simulink model "capstone_sim"  (R2021a)
settings: Solver=VariableStepAuto  StartTime=0.0  StopTime=1.5  RelTol=1e-3
values from neighbouring files (symbols this model uses):
  Jm = 500*(10^-3)*(10^-2)^2    (= 5e-05)    [capstone.m]
  Ka_cur = 1/Kp_cur    (= 521477.533066)    [capstone.m]
  Ka_spd = 1/Kp_spd    (= 8.45112747818)    [capstone.m]
  Kd_pos = Wcp/Wcs    (= 0.1)    [capstone.m]
  Ke = 0.0531    [capstone.m]
  Ki_cur = Ra * Wcc    (= 273.946879393)    [capstone.m]
  Ki_spd = Kp_spd*Wcs/5    (= 2.97389209826)    [capstone.m]
  Kp_cur = La * Wcc    (= 1.91762815575e-06)    [capstone.m]
  Kp_pos = Wcp    (= 12.5663706144)    [capstone.m]
  Kp_spd = Jm*Wcs/Ke    (= 0.118327406915)    [capstone.m]
  Kt = 0.0531    [capstone.m]
  La = 1.526*10^-9    (= 1.526e-09)    [capstone.m]
  Loadtorq = m*9.81*0.01/20    (= 0)    [capstone.m]
  max_cur = 12    [capstone.m]
  max_spd = 3000*(30/pi)    (= 28647.8897565)    [capstone.m]
  n = 20    [capstone.m]
  Ra = 0.218    [capstone.m]
  tau = 1    [capstone.m]
  wa = 10    [capstone.m]
settings Model: PacingRate=1000  Creator=syl12  LastModifiedBy=syl12

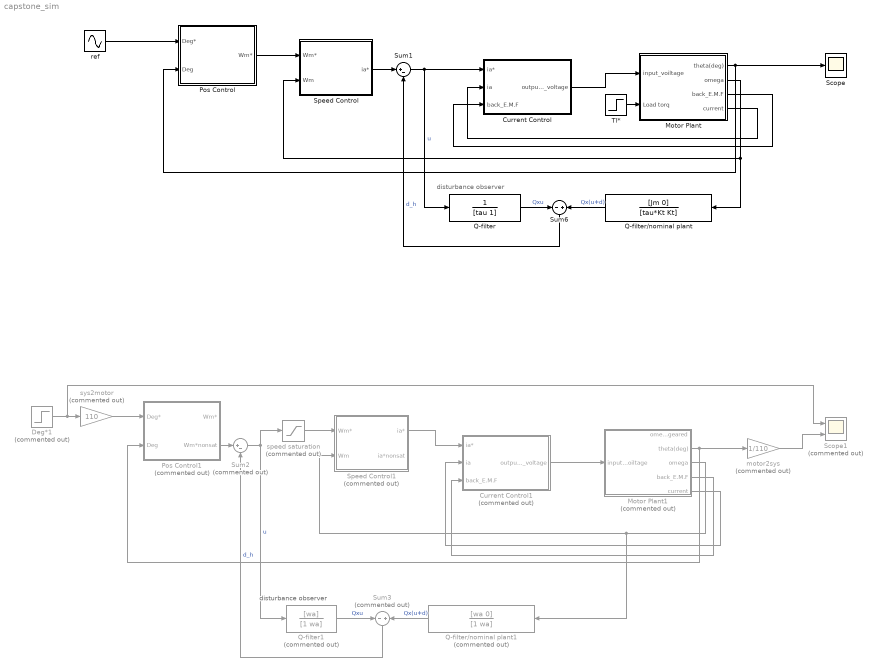
== system capstone_sim ==
  note: disturbance observer
  note: disturbance observer
  Current Control : Subsystem
  Current Control1 : Subsystem  Commented=on
  Deg*1 : Step  Commented=on  Time=0  After=5  SampleTime=0
  Motor Plant : Subsystem
  Motor Plant1 : Subsystem  Commented=on
  Pos Control : Subsystem
  Pos Control1 : Subsystem  Commented=on
  Q-filter : TransferFcn  Denominator=[tau 1]
  Q-filter/nominal plant : TransferFcn  Numerator=[Jm 0]  Denominator=[tau*Kt Kt]
  Q-filter/nominal plant1 : TransferFcn  Commented=on  Numerator=[wa 0]  Denominator=[1 wa]
  Q-filter1 : TransferFcn  Commented=on  Numerator=[wa]  Denominator=[1 wa]
  Scope : Scope
  Scope1 : Scope  Commented=on  NumInputPorts=2
  Speed Control : Subsystem
  Speed Control1 : Subsystem  Commented=on
  Sum1 : Sum  Inputs=|+-
  Sum2 : Sum  Commented=on  Inputs=|+-
  Sum3 : Sum  Commented=on  Inputs=-|+
  Sum6 : Sum  Inputs=-|+
  Tl* : Step  Time=0  After=5  SampleTime=0
  motor2sys : Gain  Commented=on  Gain=1/110
  ref : Sin  Amplitude=5  Frequency=0.15915  SampleTime=0
  speed saturation : Saturate  Commented=on  UpperLimit=max_spd*60/(2*pi*20)  LowerLimit=-max_spd*60/(2*pi*20)
  sys2motor : Gain  Commented=on  Gain=110
  wires:
  Pos Control/1(Wm*) -> Speed Control/1(Wm*)
  Speed Control/1(ia*) -> Sum1/1
  Motor Plant/4(current) -> Current Control/2(ia)
  Motor Plant/2(omega) -> Speed Control/2(Wm), Q-filter/nominal plant/1
  Motor Plant/3(back_E.M.F) -> Current Control/3(back_E.M.F)
  Q-filter/nominal plant/1 -> Sum6/2  "Qx(u+d)"
  Sum1/1 -> Current Control/1(ia*), Q-filter/1  "u"
  Current Control/1(output_voltage) -> Motor Plant/1(input_voiltage)
  Q-filter/1 -> Sum6/1  "Qxu"
  ref/1 -> Pos Control/1(Deg*)
  Motor Plant/1(theta(deg)) -> Scope/1, Pos Control/2(Deg)
  motor2sys/1 -> Scope1/2
  sys2motor/1 -> Pos Control1/1(Deg*)
  Motor Plant1/4(back_E.M.F) -> Current Control1/3(back_E.M.F)
  Motor Plant1/2(theta(deg)) -> motor2sys/1, Pos Control1/2(Deg)
  Motor Plant1/3(omega) -> Q-filter/nominal plant1/1, Speed Control1/2(Wm)
  Deg*1/1 -> Scope1/1, sys2motor/1
  Speed Control1/1(ia*) -> Current Control1/1(ia*)
  Motor Plant1/5(current) -> Current Control1/2(ia)
  Current Control1/1(output_voltage) -> Motor Plant1/1(input_voiltage)
  Q-filter/nominal plant1/1 -> Sum3/2  "Qx(u+d)"
  Q-filter1/1 -> Sum3/1  "Qxu"
  Pos Control1/2(Wm*nonsat) -> Sum2/1
  speed saturation/1 -> Speed Control1/1(Wm*)
  Sum2/1 -> speed saturation/1, Q-filter1/1  "u"
  Sum3/1 -> Sum2/2  "d_h"
  Sum6/1 -> Sum1/2  "d_h"
  Tl*/1 -> Motor Plant/2(Load torq)

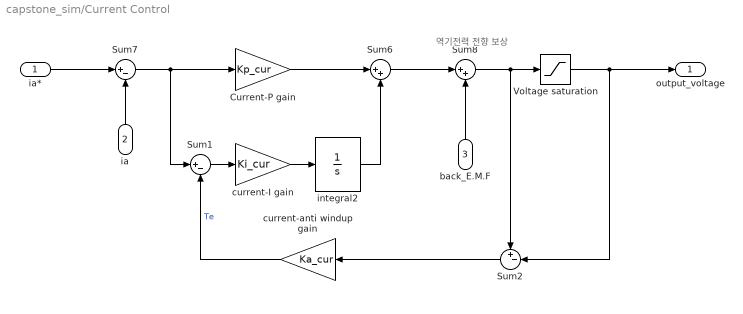
== system capstone_sim/Current Control ==
  note: 역기전력 전향 보상
  ia* : Inport
  ia : Inport  Port=2
  back_E.M.F : Inport  Port=3
  Current-P gain : Gain  Gain=Kp_cur
  Sum1 : Sum  Inputs=|+-
  Sum2 : Sum  Inputs=+-|
  Sum6 : Sum  Inputs=|++
  Sum7 : Sum  Inputs=|+-
  Sum8 : Sum  Inputs=|++
  Voltage saturation : Saturate  UpperLimit=24  LowerLimit=-24  ZeroCross=off
  current-I gain : Gain  Gain=Ki_cur
  current-anti windup gain : Gain  Gain=Ka_cur
  integral2 : TransferFcn  Denominator=[1 0]
  output_voltage : Outport
  wires:
  Sum6/1 -> Sum8/1
  ia*/1 -> Sum7/1
  integral2/1 -> Sum6/2
  Sum7/1 -> Current-P gain/1, Sum1/1
  Current-P gain/1 -> Sum6/1
  current-I gain/1 -> integral2/1
  back_E.M.F/1 -> Sum8/2
  Voltage saturation/1 -> Sum2/2, output_voltage/1
  Sum8/1 -> Sum2/1, Voltage saturation/1
  ia/1 -> Sum7/2
  Sum1/1 -> current-I gain/1
  current-anti windup gain/1 -> Sum1/2  "Te"
  Sum2/1 -> current-anti windup gain/1

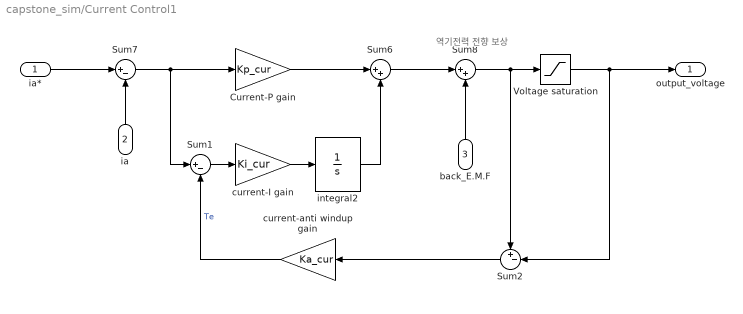
== system capstone_sim/Current Control1 ==
  note: 역기전력 전향 보상
  ia* : Inport
  ia : Inport  Port=2
  back_E.M.F : Inport  Port=3
  Current-P gain : Gain  Gain=Kp_cur
  Sum1 : Sum  Inputs=|+-
  Sum2 : Sum  Inputs=+-|
  Sum6 : Sum  Inputs=|++
  Sum7 : Sum  Inputs=|+-
  Sum8 : Sum  Inputs=|++
  Voltage saturation : Saturate  UpperLimit=24  LowerLimit=-24  ZeroCross=off
  current-I gain : Gain  Gain=Ki_cur
  current-anti windup gain : Gain  Gain=Ka_cur
  integral2 : TransferFcn  Denominator=[1 0]
  output_voltage : Outport
  wires:
  Sum6/1 -> Sum8/1
  ia*/1 -> Sum7/1
  integral2/1 -> Sum6/2
  Sum7/1 -> Current-P gain/1, Sum1/1
  Current-P gain/1 -> Sum6/1
  current-I gain/1 -> integral2/1
  back_E.M.F/1 -> Sum8/2
  Voltage saturation/1 -> Sum2/2, output_voltage/1
  Sum8/1 -> Sum2/1, Voltage saturation/1
  ia/1 -> Sum7/2
  Sum1/1 -> current-I gain/1
  current-anti windup gain/1 -> Sum1/2  "Te"
  Sum2/1 -> current-anti windup gain/1

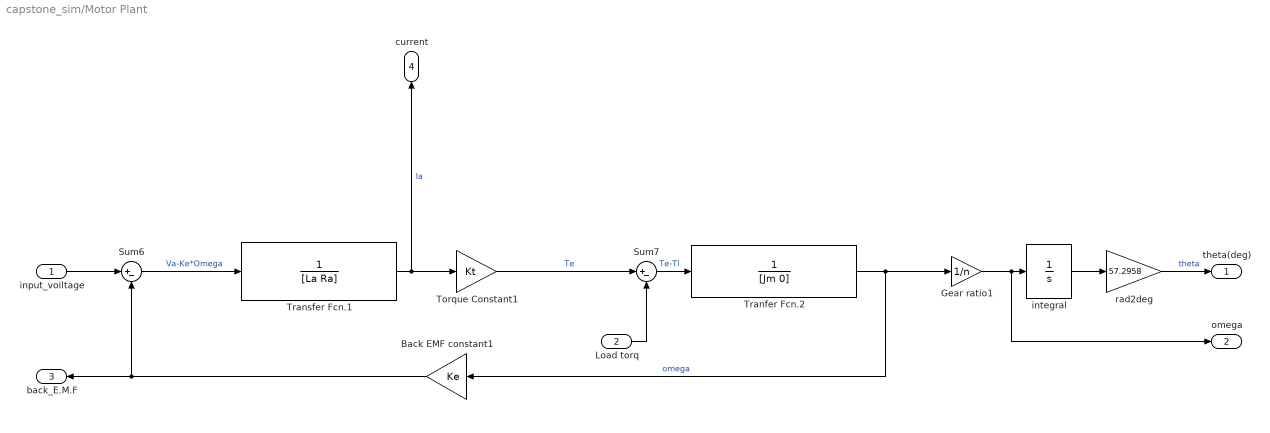
== system capstone_sim/Motor Plant ==
  input_voiltage : Inport
  Load torq : Inport  Port=2
  Back EMF constant1 : Gain  Gain=Ke
  Gear ratio1 : Gain  Gain=1/n
  Sum6 : Sum  Inputs=|+-
  Sum7 : Sum  Inputs=|+-
  Torque Constant1 : Gain  Gain=Kt
  Tranfer Fcn.2 : TransferFcn  Denominator=[Jm 0]
  Transfer Fcn.1 : TransferFcn  Denominator=[La Ra]
  integral : TransferFcn  Denominator=[1 0]
  rad2deg : Gain  Gain=57.2958
  theta(deg) : Outport
  omega : Outport  Port=2
  back_E.M.F : Outport  Port=3
  current : Outport  Port=4
  wires:
  Sum6/1 -> Transfer Fcn.1/1  "Va-Ke*Omega"
  Tranfer Fcn.2/1 -> Gear ratio1/1, Back EMF constant1/1  "omega"
  Sum7/1 -> Tranfer Fcn.2/1  "Te-Tl"
  Back EMF constant1/1 -> back_E.M.F/1, Sum6/2
  input_voiltage/1 -> Sum6/1
  Transfer Fcn.1/1 -> Torque Constant1/1, current/1  "Ia"
  integral/1 -> rad2deg/1
  rad2deg/1 -> theta(deg)/1  "theta"
  Gear ratio1/1 -> omega/1, integral/1
  Torque Constant1/1 -> Sum7/1  "Te"
  Load torq/1 -> Sum7/2

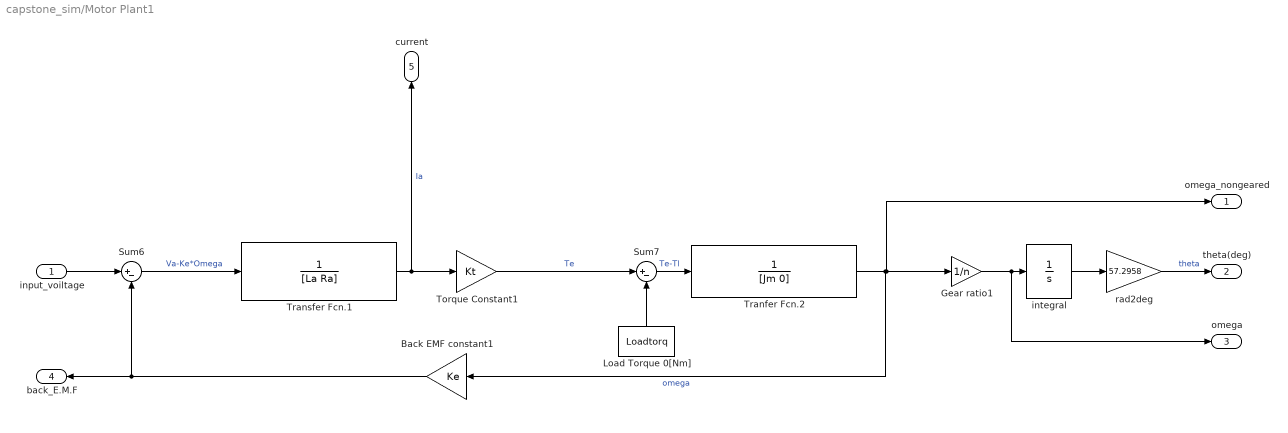
== system capstone_sim/Motor Plant1 ==
  input_voiltage : Inport
  Back EMF constant1 : Gain  Gain=Ke
  Gear ratio1 : Gain  Gain=1/n
  Load Torque 0[Nm] : Constant  Value=Loadtorq
  Sum6 : Sum  Inputs=|+-
  Sum7 : Sum  Inputs=|+-
  Torque Constant1 : Gain  Gain=Kt
  Tranfer Fcn.2 : TransferFcn  Denominator=[Jm 0]
  Transfer Fcn.1 : TransferFcn  Denominator=[La Ra]
  integral : TransferFcn  Denominator=[1 0]
  rad2deg : Gain  Gain=57.2958
  omega_nongeared : Outport
  theta(deg) : Outport  Port=2
  omega : Outport  Port=3
  back_E.M.F : Outport  Port=4
  current : Outport  Port=5
  wires:
  Sum6/1 -> Transfer Fcn.1/1  "Va-Ke*Omega"
  Tranfer Fcn.2/1 -> omega_nongeared/1, Gear ratio1/1, Back EMF constant1/1  "omega"
  Sum7/1 -> Tranfer Fcn.2/1  "Te-Tl"
  Back EMF constant1/1 -> back_E.M.F/1, Sum6/2
  input_voiltage/1 -> Sum6/1
  Transfer Fcn.1/1 -> Torque Constant1/1, current/1  "Ia"
  integral/1 -> rad2deg/1
  rad2deg/1 -> theta(deg)/1  "theta"
  Gear ratio1/1 -> omega/1, integral/1
  Torque Constant1/1 -> Sum7/1  "Te"
  Load Torque 0[Nm]/1 -> Sum7/2

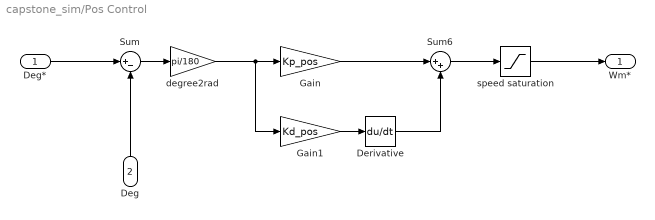
== system capstone_sim/Pos Control ==
  Deg* : Inport
  Deg : Inport  Port=2
  Derivative : Derivative
  Gain : Gain  Gain=Kp_pos
  Gain1 : Gain  Gain=Kd_pos
  Sum : Sum  Inputs=|+-
  Sum6 : Sum  Inputs=|++
  degree2rad : Gain  Gain=pi/180
  speed saturation : Saturate  UpperLimit=max_spd*60/(2*pi*20)  LowerLimit=-max_spd*60/(2*pi*20)
  Wm* : Outport
  wires:
  Derivative/1 -> Sum6/2
  Deg*/1 -> Sum/1
  speed saturation/1 -> Wm*/1
  Gain/1 -> Sum6/1
  Sum6/1 -> speed saturation/1
  Deg/1 -> Sum/2
  Gain1/1 -> Derivative/1
  Sum/1 -> degree2rad/1
  degree2rad/1 -> Gain1/1, Gain/1

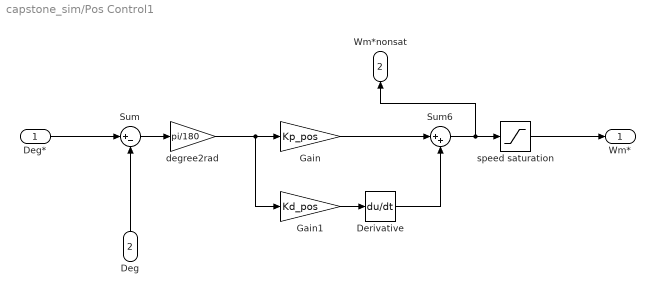
== system capstone_sim/Pos Control1 ==
  Deg* : Inport
  Deg : Inport  Port=2
  Derivative : Derivative
  Gain : Gain  Gain=Kp_pos
  Gain1 : Gain  Gain=Kd_pos
  Sum : Sum  Inputs=|+-
  Sum6 : Sum  Inputs=|++
  degree2rad : Gain  Gain=pi/180
  speed saturation : Saturate  UpperLimit=max_spd*60/(2*pi*20)  LowerLimit=-max_spd*60/(2*pi*20)
  Wm* : Outport
  Wm*nonsat : Outport  Port=2
  wires:
  Derivative/1 -> Sum6/2
  Deg*/1 -> Sum/1
  speed saturation/1 -> Wm*/1
  Gain/1 -> Sum6/1
  Sum6/1 -> speed saturation/1, Wm*nonsat/1
  Deg/1 -> Sum/2
  Gain1/1 -> Derivative/1
  Sum/1 -> degree2rad/1
  degree2rad/1 -> Gain1/1, Gain/1

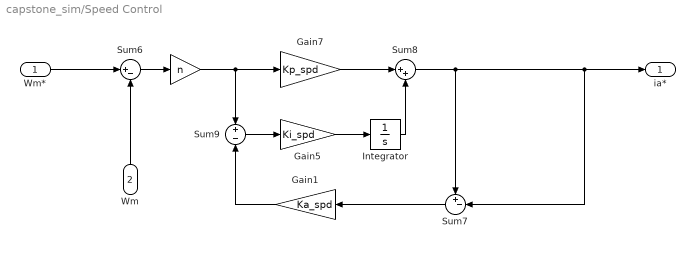
== system capstone_sim/Speed Control ==
  Wm* : Inport
  Wm : Inport  Port=2
  " " : Gain  Gain=n
  Gain1 : Gain  Gain=Ka_spd
  Gain5 : Gain  Gain=Ki_spd
  Gain7 : Gain  Gain=Kp_spd
  Integrator : Integrator
  Sum6 : Sum  Inputs=|+-
  Sum7 : Sum  Inputs=+-|
  Sum8 : Sum  Inputs=|++
  Sum9 : Sum  Inputs=+|-
  ia* : Outport
  wires:
  Gain5/1 -> Integrator/1
  Sum8/1 -> Sum7/2, ia*/1, Sum7/1
  Wm/1 -> Sum6/2
  Gain1/1 -> Sum9/2
  Integrator/1 -> Sum8/2
  " "/1 -> Gain7/1, Sum9/1
  Sum6/1 -> " "/1
  Sum7/1 -> Gain1/1
  Gain7/1 -> Sum8/1
  Wm*/1 -> Sum6/1
  Sum9/1 -> Gain5/1

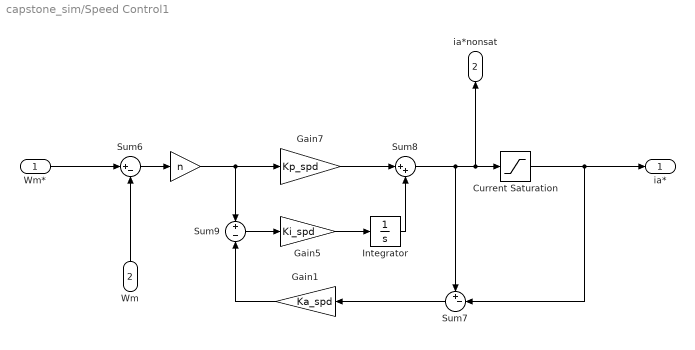
== system capstone_sim/Speed Control1 ==
  Wm* : Inport
  Wm : Inport  Port=2
  " " : Gain  Gain=n
  Current Saturation : Saturate  UpperLimit=max_cur  LowerLimit=-max_cur  ZeroCross=off
  Gain1 : Gain  Gain=Ka_spd
  Gain5 : Gain  Gain=Ki_spd
  Gain7 : Gain  Gain=Kp_spd
  Integrator : Integrator
  Sum6 : Sum  Inputs=|+-
  Sum7 : Sum  Inputs=+-|
  Sum8 : Sum  Inputs=|++
  Sum9 : Sum  Inputs=+|-
  ia* : Outport
  ia*nonsat : Outport  Port=2
  wires:
  Gain5/1 -> Integrator/1
  Sum8/1 -> Current Saturation/1, ia*nonsat/1, Sum7/1
  Current Saturation/1 -> Sum7/2, ia*/1
  Wm/1 -> Sum6/2
  Gain1/1 -> Sum9/2
  Integrator/1 -> Sum8/2
  " "/1 -> Gain7/1, Sum9/1
  Sum6/1 -> " "/1
  Sum7/1 -> Gain1/1
  Gain7/1 -> Sum8/1
  Wm*/1 -> Sum6/1
  Sum9/1 -> Gain5/1
